simulink model "Vending_Machine_Mealy"  (R2016a)
settings: Solver=VariableStepAuto  StartTime=0.0  StopTime=100.0  RelTol=1e-3
model workspace (MAT data in the model file):
  choice = Simulink.Parameter
  choice.Value = 0
  choice.DataType = 'auto'
  choice.Min = 0
  choice.Max = 3
  choice.Dimensions = [1 1]
  sw = 1
settings Model: Creator=Admin  LastModifiedBy=Admin

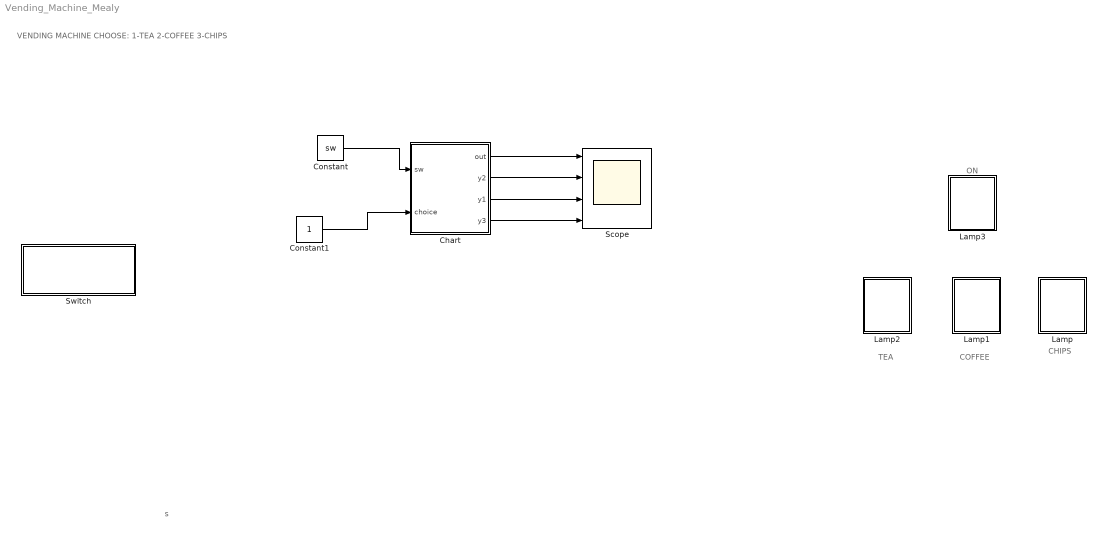
== system Vending_Machine_Mealy ==
  note: s
  note: VENDING MACHINE
      |
      | CHOOSE:
      |
      | 1-TEA
      | 2-COFFEE
      | 3-CHIPS
  note: CHIPS
  note: COFFEE
  note: TEA
  note: ON
  Chart : Stateflow chart  TreatAsAtomicUnit=on
  Constant : Constant  Value=sw
  Constant1 : Constant
  Lamp : Subsystem  DialogController=hmiCreateDDGDialog  IsWebBlock=on  mask(MWDashboardBlock){webBlockId=00d03fe9-44a6-4e09-90a4-3ba281b09aed, webBlockType=lamp, ShowInLibBrowser=on, ShowInitialText=on, HMISrcModelName=Vending_Machine_Mealy}
      mask prompts: webBlockType "WebBlock Type"; HMISrcModelName "Source Model"
      mask Help: helpview([docroot '/mapfiles/simulink.map'], 'hmi_lamp')
      mask Display:
      | if strcmp(get_param(bdroot(gcb),'BlockDiagramType'), 'library')
      |     image([(matlabroot) '/toolbox/simulink/hmi/icons/Lamp.png']);
      | end
  Lamp1 : Subsystem  DialogController=hmiCreateDDGDialog  IsWebBlock=on  mask(MWDashboardBlock){webBlockId=cda5c25e-f60c-4207-a728-e7031f7584b7, webBlockType=lamp, ShowInLibBrowser=on, ShowInitialText=on, HMISrcModelName=Vending_Machine_Mealy}
      mask prompts: webBlockType "WebBlock Type"; HMISrcModelName "Source Model"
      mask Help: helpview([docroot '/mapfiles/simulink.map'], 'hmi_lamp')
      mask Display:
      | if strcmp(get_param(bdroot(gcb),'BlockDiagramType'), 'library')
      |     image([(matlabroot) '/toolbox/simulink/hmi/icons/Lamp.png']);
      | end
  Lamp2 : Subsystem  DialogController=hmiCreateDDGDialog  IsWebBlock=on  mask(MWDashboardBlock){webBlockId=b2c77429-8ef9-4fa6-baef-71650182eb19, webBlockType=lamp, ShowInLibBrowser=on, ShowInitialText=on, HMISrcModelName=Vending_Machine_Mealy}
      mask prompts: webBlockType "WebBlock Type"; HMISrcModelName "Source Model"
      mask Help: helpview([docroot '/mapfiles/simulink.map'], 'hmi_lamp')
      mask Display:
      | if strcmp(get_param(bdroot(gcb),'BlockDiagramType'), 'library')
      |     image([(matlabroot) '/toolbox/simulink/hmi/icons/Lamp.png']);
      | end
  Lamp3 : Subsystem  DialogController=hmiCreateDDGDialog  IsWebBlock=on  mask(MWDashboardBlock){webBlockId=2ef2be1a-4d03-4c4a-929d-ac159d21a6f1, webBlockType=lamp, ShowInLibBrowser=on, ShowInitialText=on, HMISrcModelName=Vending_Machine_Mealy}
      mask prompts: webBlockType "WebBlock Type"; HMISrcModelName "Source Model"
      mask Help: helpview([docroot '/mapfiles/simulink.map'], 'hmi_lamp')
      mask Display:
      | if strcmp(get_param(bdroot(gcb),'BlockDiagramType'), 'library')
      |     image([(matlabroot) '/toolbox/simulink/hmi/icons/Lamp.png']);
      | end
  Scope : Scope  NumInputPorts=4
  "Switch " : Subsystem  DialogController=hmiCreateDDGDialog  IsWebBlock=on  mask(MWDashboardBlock){webBlockId=d6880685-53ef-45f7-bc64-ff5739e381f5, webBlockType=sliderswitch, ShowInLibBrowser=on, ShowInitialText=on, HMISrcModelName=Vending_Machine_Mealy}
      mask prompts: webBlockId "WebBlock Id"; webBlockType "WebBlock Type"; HMISrcModelName "Source Model"
      mask Help: helpview([docroot '/mapfiles/simulink.map'], 'hmi_slider_switch')
      mask Display:
      | if strcmp(get_param(bdroot(gcb),'BlockDiagramType'), 'library')
      |     image([(matlabroot) '/toolbox/simulink/hmi/icons/SliderSwitch.png']);
      | end
  wires:
  Chart/1(out) -> Scope/1
  Chart/2(y2) -> Scope/2
  Chart/3(y1) -> Scope/3
  Chart/4(y3) -> Scope/4
  Constant/1 -> Chart/1(sw)
  Constant1/1 -> Chart/2(choice)

== system Vending_Machine_Mealy/Lamp ==

== system Vending_Machine_Mealy/Lamp1 ==

== system Vending_Machine_Mealy/Lamp2 ==

== system Vending_Machine_Mealy/Lamp3 ==

== system Vending_Machine_Mealy/Switch  ==

== stateflow chart Vending_Machine_Mealy/Chart ==
  state Main
    entry:
    during:
    exit:
  state Tea
    entry:
    during:
    exit:
  state Enable_logic
    entry:
    during:
    exit:
  state Chips_
    entry:
    disp('chips');
    during:
    exit:
  state Coffee
    entry:
    during:
    exit:
  (default) -> Enable_logic
  Enable_logic -> Main : [sw==1]
      | {out=1;
      | out=1;
      | y1=0;
      | y2=0;
      | y3=0;}
  Main -> Tea [order 2] : [choice==1]
      | {out=1;
      | y1=1;
      | y2=0;
      | y3=0;}
  Main -> Enable_logic [order 1] : [sw==0]
      |
      | {out=0;
      | y1=0;
      | y2=0;
      | y3=0;}
  Coffee -> Enable_logic [order 1] : [sw==0]
      |
      | {out=0;}
  Tea -> Main : [after(10,tick)]
      | {out=1;
      | y1=0;
      | y2=0;
      | y3=0;}
  Coffee -> Main [order 2] : [after(10,tick)]
      | {out=1;
      | y1=0;
      | y2=0;
      | y3=0;}
  Main -> Coffee [order 4] : [choice==2]
      | {out=1;
      | y1=0;
      | y2=1;
      | y3=0;}
  Main -> Chips_ [order 3] : [choice==3]
      | {out=1;
      | y1=0;
      | y2=0;
      | y3=1;}
  Chips_ -> Main : [after(20,tick)]
      | {out=1;
      | y1=0;
      | y2=0;
      | y3=0;}
  data: sw input; choice input; out output; y2 output; y1 output; y3 output
